simulink model "SpeedSensingBasedOnHallSensors"  (R2017b)
settings: Solver=ode5  StartTime=0.0  StopTime=2  FixedStep=0.000001  RelTol=1e-3
libraries: simulink x4
settings Model: Creator=uidp7521  LastModifiedBy=uidp7521

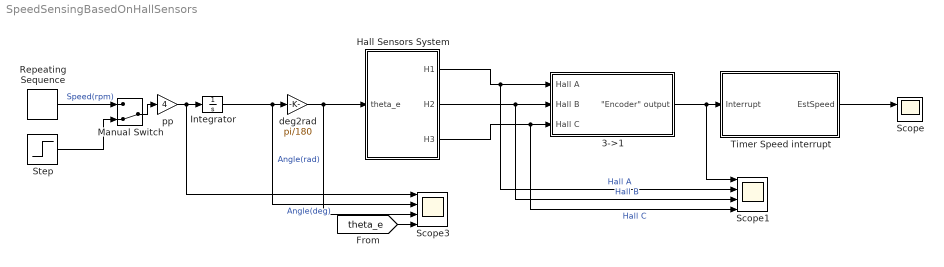
== system SpeedSensingBasedOnHallSensors ==
  3->1 : Subsystem
  Hall Sensors System : Subsystem
  Integrator : Integrator
  Manual Switch : ManualSwitch  CurrentSetting=0
  Repeating Sequence : simulink/Sources/Repeating Sequence  rep_seq_t=[0 1 2]  rep_seq_y=[0 1000 0]
  Scope : Scope  NumInputPorts=2
  Scope1 : Scope  NumInputPorts=4
  Scope3 : Scope  NumInputPorts=4
  Step : Step  Time=0.1  After=600  SampleTime=0
  Timer Speed interrupt : Subsystem
  deg2rad : Gain  Gain=pi/180
  pp : Gain  Gain=4
  wires:
  Hall Sensors System/2(H2) -> Scope1/3, 3->1/2(Hall B)  "Hall B"
  Hall Sensors System/1(H1) -> 3->1/1(Hall A), Scope1/2  "Hall A"
  Hall Sensors System/3(H3) -> Scope1/4, 3->1/3(Hall C)  "Hall C"
  Integrator/1 -> Scope3/2, deg2rad/1  "Angle(deg)"
  deg2rad/1 -> Scope3/3, Hall Sensors System/1(theta_e)  "Angle(rad)"
  3->1/1("\"Encoder\" output") -> Scope1/1, Timer Speed interrupt/1(Interrupt)
  Timer Speed interrupt/1(EstSpeed) -> Scope/1
  [theta_e] -> Scope3/4
  pp/1 -> Scope3/1, Integrator/1
  Manual Switch/1 -> pp/1
  Repeating Sequence/1 -> Manual Switch/1  "Speed(rpm)"
  Step/1 -> Manual Switch/2

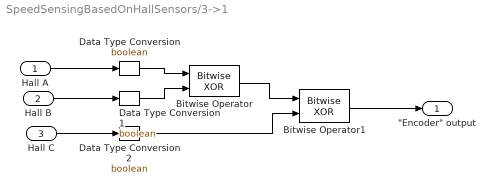
== system SpeedSensingBasedOnHallSensors/3->1 ==
  Hall A : Inport
  Hall B : Inport  Port=2
  Hall C : Inport  Port=3
  Bitwise Operator : simulink/Logic and Bit Operations/Bitwise Operator  logicop=XOR  UseBitMask=off  NumInputPorts=2  BitMask=bin2dec('11011001')  BitMaskRealWorld=Stored Integer
  Bitwise Operator1 : simulink/Logic and Bit Operations/Bitwise Operator  logicop=XOR  UseBitMask=off  NumInputPorts=2  BitMask=bin2dec('11011001')  BitMaskRealWorld=Stored Integer
  Data Type Conversion : DataTypeConversion  OutDataTypeStr=boolean
  Data Type Conversion1 : DataTypeConversion  OutDataTypeStr=boolean
  Data Type Conversion2 : DataTypeConversion  OutDataTypeStr=boolean
  "\"Encoder\" output" : Outport
  wires:
  Data Type Conversion1/1 -> Bitwise Operator/2
  Data Type Conversion/1 -> Bitwise Operator/1
  Hall B/1 -> Data Type Conversion1/1
  Hall C/1 -> Data Type Conversion2/1
  Hall A/1 -> Data Type Conversion/1
  Data Type Conversion2/1 -> Bitwise Operator1/2
  Bitwise Operator/1 -> Bitwise Operator1/1
  Bitwise Operator1/1 -> "\"Encoder\" output"/1

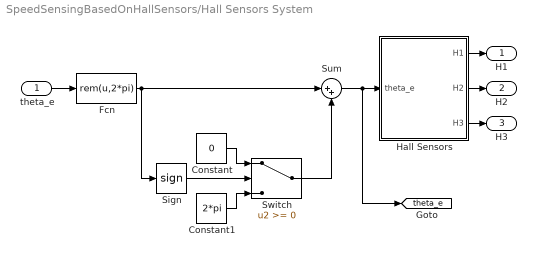
== system SpeedSensingBasedOnHallSensors/Hall Sensors System ==
  theta_e : Inport
  Constant : Constant  Value=0
  Constant1 : Constant  Value=2*pi
  Fcn : Fcn  Expr=rem(u,2*pi)
  Hall Sensors : Subsystem
  Sign : Signum
  Sum : Sum  Inputs=|++
  Switch : Switch
  H1 : Outport
  H2 : Outport  Port=2
  H3 : Outport  Port=3
  tag scope: theta_e=global
  wires:
  Hall Sensors/3("H3 ") -> H3/1
  Hall Sensors/1("H1 ") -> H1/1
  Hall Sensors/2("H2 ") -> H2/1
  theta_e/1 -> Fcn/1
  Fcn/1 -> Sum/1, Sign/1
  Sign/1 -> Switch/2
  Constant1/1 -> Switch/3
  Switch/1 -> Sum/2
  Sum/1 -> [theta_e], Hall Sensors/1(theta_e)
  Constant/1 -> Switch/1

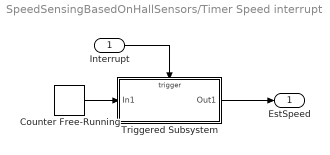
== system SpeedSensingBasedOnHallSensors/Timer Speed interrupt ==
  Interrupt : Inport
  Counter Free-Running : simulink/Sources/Counter Free-Running  NumBits=16  tsamp=0.000001
  Triggered Subsystem : Subsystem  TreatAsAtomicUnit=on
  EstSpeed : Outport
  wires:
  Triggered Subsystem/1(Out1) -> EstSpeed/1
  Counter Free-Running/1 -> Triggered Subsystem/1(In1)
  Interrupt/1 -> Triggered Subsystem/Trigger

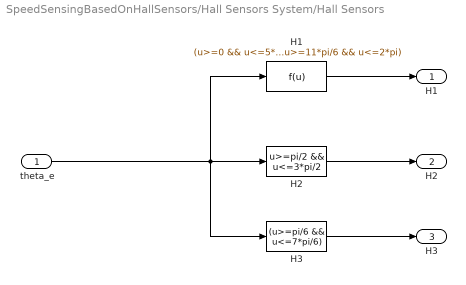
== system SpeedSensingBasedOnHallSensors/Hall Sensors System/Hall Sensors ==
  theta_e : Inport
  H1 : Fcn  Expr=(u>=0 && u<=5*pi/6) || (u>=11*pi/6 && u<=2*pi)
  H2 : Fcn  Expr=u>=pi/2 && u<=3*pi/2
  H3 : Fcn  Expr=(u>=pi/6 && u<=7*pi/6)
  "H1 " : Outport
  "H2 " : Outport  Port=2
  "H3 " : Outport  Port=3
  wires:
  theta_e/1 -> H3/1, H1/1, H2/1
  H1/1 -> "H1 "/1
  H2/1 -> "H2 "/1
  H3/1 -> "H3 "/1

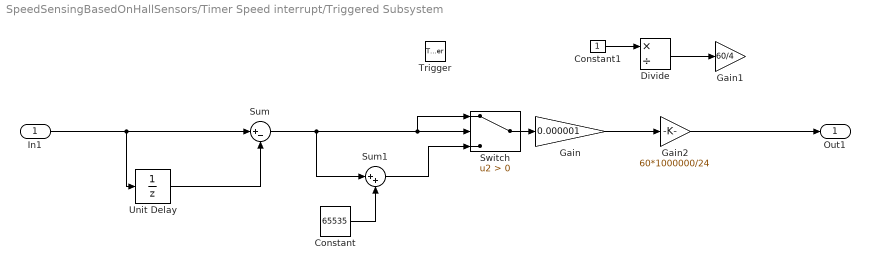
== system SpeedSensingBasedOnHallSensors/Timer Speed interrupt/Triggered Subsystem ==
  In1 : Inport
  Trigger : TriggerPort  TriggerType=either  VariantControl=Variant
  Constant : Constant  Value=65535
  Constant1 : Constant
  Divide : Product  Inputs=*/
  Gain : Gain  Gain=0.000001
  Gain1 : Gain  Gain=60/4
  Gain2 : Gain  Gain=60*1000000/24
  Sum : Sum  Inputs=|+-
  Sum1 : Sum  Inputs=|++
  Switch : Switch  Criteria=u2 > Threshold
  Unit Delay : UnitDelay  SampleTime=-1
  Out1 : Outport
  wires:
  In1/1 -> Unit Delay/1, Sum/1
  Unit Delay/1 -> Sum/2
  Sum/1 -> Switch/1, Switch/2, Sum1/1
  Constant/1 -> Sum1/2
  Sum1/1 -> Switch/3
  Switch/1 -> Gain/1
  Divide/1 -> Gain1/1
  Constant1/1 -> Divide/1
  Gain2/1 -> Out1/1
  Gain/1 -> Gain2/1
